simulink model "model2"  (R2021a)
settings: Solver=VariableStepAuto  StartTime=0.0  StopTime=2  RelTol=1e-3
model workspace (MAT data in the model file):
  B = 4.6752e-05
  J = 2.0095e-05
  Ld = 0.0078
  Lq = 0.0078
  P = 4
  Rs = 1.2
  lambda = 0.154
settings Model: Creator=Sreejith  LastModifiedBy=Sreejith

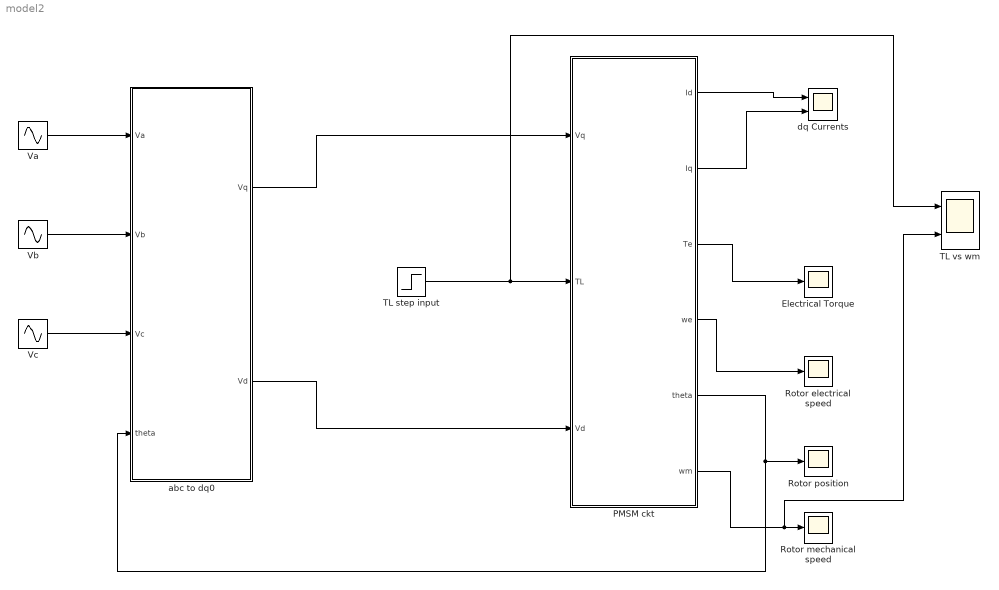
== system model2 ==
  Electrical Torque : Scope
  PMSM ckt : Subsystem
  Rotor electrical speed : Scope
  Rotor mechanical speed : Scope
  Rotor position : Scope
  TL step input : Step  Before=1  After=2  SampleTime=0
  TL vs wm : Scope  NumInputPorts=2
  Va : Sin  Amplitude=220*sqrt(2)  Frequency=100*pi  SampleTime=0
  Vb : Sin  Amplitude=220*sqrt(2)  Frequency=100*pi  Phase=-2*pi/3  SampleTime=0
  Vc : Sin  Amplitude=220*sqrt(2)  Frequency=100*pi  Phase=2*pi/3  SampleTime=0
  abc to dq0 : Subsystem
  dq Currents : Scope  NumInputPorts=2
  wires:
  abc to dq0/1(Vq) -> PMSM ckt/1(Vq)
  TL step input/1 -> TL vs wm/1, PMSM ckt/2(TL)
  abc to dq0/2(Vd) -> PMSM ckt/3(Vd)
  PMSM ckt/1(Id) -> dq Currents/1
  PMSM ckt/2(Iq) -> dq Currents/2
  PMSM ckt/3(Te) -> Electrical Torque/1
  PMSM ckt/4(we) -> Rotor electrical speed/1
  PMSM ckt/5(theta) -> abc to dq0/4(theta), Rotor position/1
  Va/1 -> abc to dq0/1(Va)
  Vb/1 -> abc to dq0/2(Vb)
  Vc/1 -> abc to dq0/3(Vc)
  PMSM ckt/6(wm) -> TL vs wm/2, Rotor mechanical speed/1

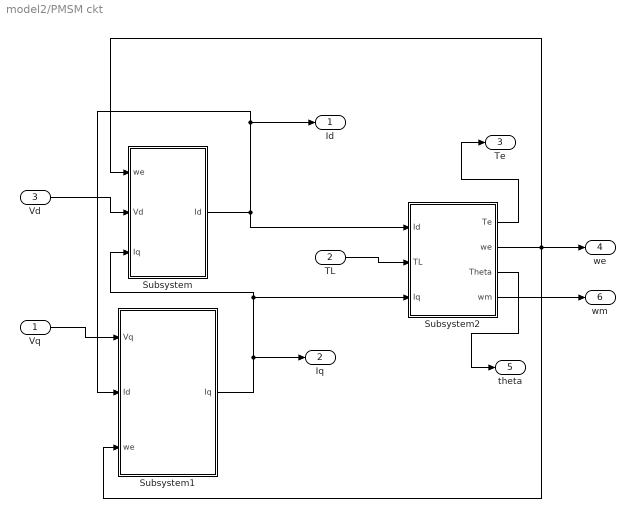
== system model2/PMSM ckt ==
  Vq : Inport
  TL : Inport  Port=2
  Vd : Inport  Port=3
  Subsystem : Subsystem
  Subsystem1 : Subsystem
  Subsystem2 : Subsystem
  Id : Outport
  Iq : Outport  Port=2
  Te : Outport  Port=3
  we : Outport  Port=4
  theta : Outport  Port=5
  wm : Outport  Port=6
  wires:
  Subsystem/1(Id) -> Id/1, Subsystem1/2(Id), Subsystem2/1(Id)
  Subsystem1/1(Iq) -> Subsystem/3(Iq), Subsystem2/3(Iq), Iq/1
  Subsystem2/1(Te) -> Te/1
  Subsystem2/2(we) -> Subsystem1/3(we), we/1, Subsystem/1(we)
  Subsystem2/3(Theta) -> theta/1
  TL/1 -> Subsystem2/2(TL)
  Vq/1 -> Subsystem1/1(Vq)
  Vd/1 -> Subsystem/2(Vd)
  Subsystem2/4(wm) -> wm/1

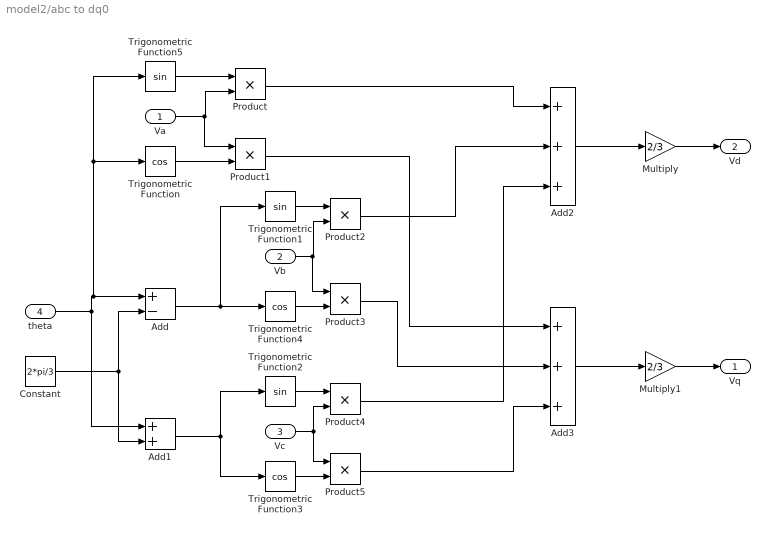
== system model2/abc to dq0 ==
  Va : Inport
  Vb : Inport  Port=2
  Vc : Inport  Port=3
  theta : Inport  Port=4
  Add : Sum  Inputs=+-
  Add1 : Sum
  Add2 : Sum  Inputs=+++
  Add3 : Sum  Inputs=+++
  Constant : Constant  Value=2*pi/3
  Multiply : Gain  Gain=2/3
  Multiply1 : Gain  Gain=2/3
  Product{,1..5} (6 alike) : Product
  Trigonometric Function : Trigonometry  Operator=cos
  Trigonometric Function1 : Trigonometry
  Trigonometric Function2 : Trigonometry
  Trigonometric Function3 : Trigonometry  Operator=cos
  Trigonometric Function4 : Trigonometry  Operator=cos
  Trigonometric Function5 : Trigonometry
  Vq : Outport
  Vd : Outport  Port=2
  wires:
  theta/1 -> Add1/1, Add/1, Trigonometric Function5/1, Trigonometric Function/1
  Constant/1 -> Add/2, Add1/2
  Add/1 -> Trigonometric Function4/1, Trigonometric Function1/1
  Add1/1 -> Trigonometric Function2/1, Trigonometric Function3/1
  Trigonometric Function5/1 -> Product/1
  Va/1 -> Product1/1, Product/2
  Trigonometric Function/1 -> Product1/2
  Trigonometric Function1/1 -> Product2/1
  Vb/1 -> Product3/1, Product2/2
  Trigonometric Function4/1 -> Product3/2
  Trigonometric Function3/1 -> Product5/2
  Trigonometric Function2/1 -> Product4/1
  Vc/1 -> Product5/1, Product4/2
  Product/1 -> Add2/1
  Product2/1 -> Add2/2
  Product4/1 -> Add2/3
  Product1/1 -> Add3/1
  Product3/1 -> Add3/2
  Product5/1 -> Add3/3
  Add2/1 -> Multiply/1
  Multiply/1 -> Vd/1
  Add3/1 -> Multiply1/1
  Multiply1/1 -> Vq/1

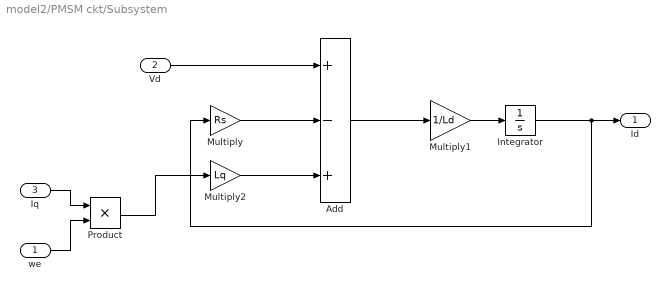
== system model2/PMSM ckt/Subsystem ==
  we : Inport
  Vd : Inport  Port=2
  Iq : Inport  Port=3
  Add : Sum  Inputs=+-+
  Integrator : Integrator
  Multiply : Gain  Gain=Rs
  Multiply1 : Gain  Gain=1/Ld
  Multiply2 : Gain  Gain=Lq
  Product : Product
  Id : Outport
  wires:
  Vd/1 -> Add/1
  Add/1 -> Multiply1/1
  Multiply1/1 -> Integrator/1
  Integrator/1 -> Multiply/1, Id/1
  Multiply/1 -> Add/2
  Iq/1 -> Product/1
  we/1 -> Product/2
  Product/1 -> Multiply2/1
  Multiply2/1 -> Add/3

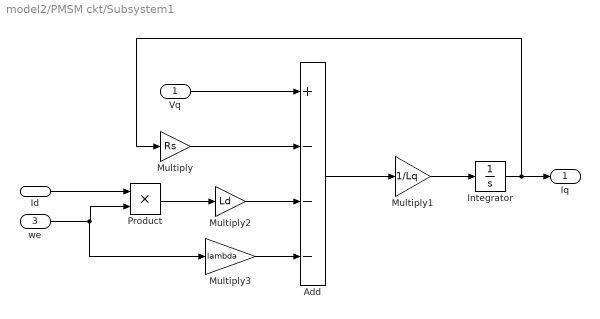
== system model2/PMSM ckt/Subsystem1 ==
  Vq : Inport
  Id : Inport  Port=2
  we : Inport  Port=3
  Add : Sum  Inputs=+---
  Integrator : Integrator
  Multiply : Gain  Gain=Rs
  Multiply1 : Gain  Gain=1/Lq
  Multiply2 : Gain  Gain=Ld
  Multiply3 : Gain  Gain=lambda
  Product : Product
  Iq : Outport
  wires:
  Vq/1 -> Add/1
  Multiply/1 -> Add/2
  Integrator/1 -> Multiply/1, Iq/1
  Add/1 -> Multiply1/1
  Multiply1/1 -> Integrator/1
  Id/1 -> Product/1
  we/1 -> Multiply3/1, Product/2
  Product/1 -> Multiply2/1
  Multiply2/1 -> Add/3
  Multiply3/1 -> Add/4

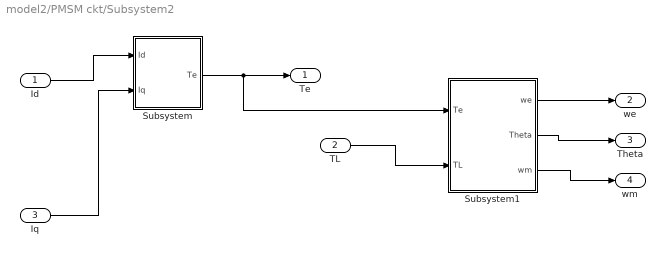
== system model2/PMSM ckt/Subsystem2 ==
  Id : Inport
  TL : Inport  Port=2
  Iq : Inport  Port=3
  Subsystem : Subsystem
  Subsystem1 : Subsystem
  Te : Outport
  we : Outport  Port=2
  Theta : Outport  Port=3
  wm : Outport  Port=4
  wires:
  Id/1 -> Subsystem/1(Id)
  Iq/1 -> Subsystem/2(Iq)
  Subsystem/1(Te) -> Subsystem1/1(Te), Te/1
  TL/1 -> Subsystem1/2(TL)
  Subsystem1/1(we) -> we/1
  Subsystem1/2(Theta) -> Theta/1
  Subsystem1/3(wm) -> wm/1

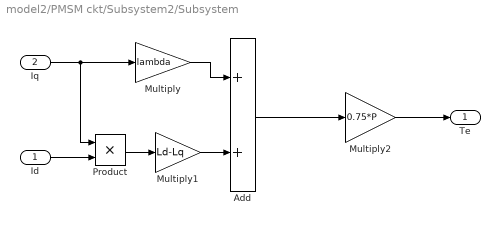
== system model2/PMSM ckt/Subsystem2/Subsystem ==
  Id : Inport
  Iq : Inport  Port=2
  Add : Sum
  Multiply : Gain  Gain=lambda
  Multiply1 : Gain  Gain=Ld-Lq
  Multiply2 : Gain  Gain=0.75*P
  Product : Product
  Te : Outport
  wires:
  Iq/1 -> Product/1, Multiply/1
  Multiply/1 -> Add/1
  Id/1 -> Product/2
  Multiply1/1 -> Add/2
  Product/1 -> Multiply1/1
  Add/1 -> Multiply2/1
  Multiply2/1 -> Te/1

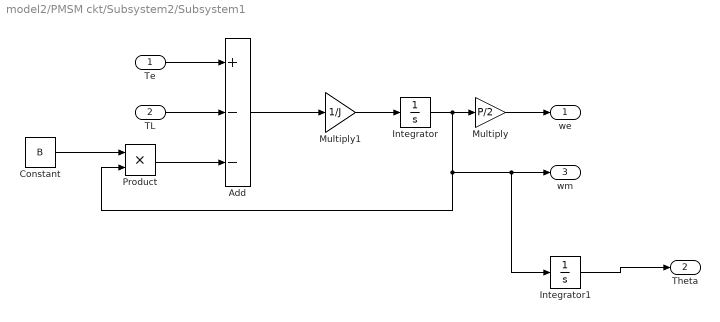
== system model2/PMSM ckt/Subsystem2/Subsystem1 ==
  Te : Inport
  TL : Inport  Port=2
  Add : Sum  Inputs=+--
  Constant : Constant  Value=B
  Integrator : Integrator
  Integrator1 : Integrator  WrapState=on  WrappedStateUpperValue=2*pi  WrappedStateLowerValue=0
  Multiply : Gain  Gain=P/2
  Multiply1 : Gain  Gain=1/J
  Product : Product
  we : Outport
  Theta : Outport  Port=2
  wm : Outport  Port=3
  wires:
  Multiply/1 -> we/1
  Multiply1/1 -> Integrator/1
  Te/1 -> Add/1
  TL/1 -> Add/2
  Product/1 -> Add/3
  Constant/1 -> Product/1
  Add/1 -> Multiply1/1
  Integrator/1 -> Product/2, Integrator1/1, wm/1, Multiply/1
  Integrator1/1 -> Theta/1
